simulink model "CS637Assignment3_1"  (R2022a)
settings: Solver=VariableStepAuto  StartTime=0.0  StopTime=5.0  RelTol=1e-3
model workspace (MAT data in the model file):
  I = 3.88e-07
  Kb = 0.000275
  Kt = 0.0059
  L = 0.00011
  R = 1.71
  b = 0
settings Model: Creator=kaush  LastModifiedBy=kaush

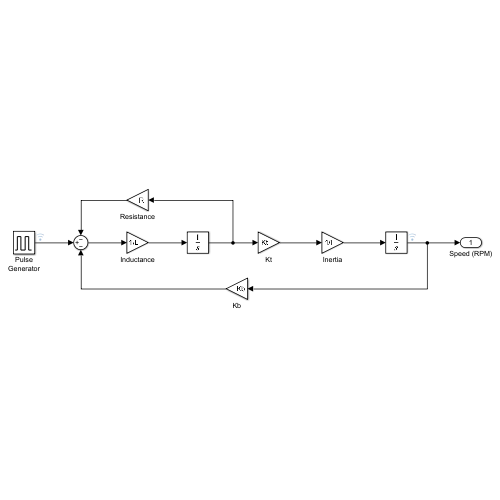
[thumbnail: Simulink's stored preview of the top-level diagram]
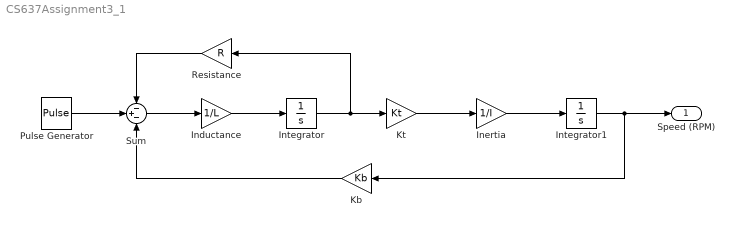
== system CS637Assignment3_1 ==
  Inductance : Gain  Gain=1/L
  Inertia : Gain  Gain=1/I
  Integrator : Integrator
  Integrator1 : Integrator
  Kb : Gain  Gain=Kb
  Kt : Gain  Gain=Kt
  Pulse Generator : DiscretePulseGenerator  PulseType=Time based  Period=0.001  PulseWidth=10
  Resistance : Gain  Gain=R
  Sum : Sum  Inputs=-+-
  Speed (RPM) : Outport
  wires:
  Kt/1 -> Inertia/1
  Inertia/1 -> Integrator1/1
  Sum/1 -> Inductance/1
  Inductance/1 -> Integrator/1
  Integrator1/1 -> Speed (RPM)/1, Kb/1
  Integrator/1 -> Kt/1, Resistance/1
  Kb/1 -> Sum/3
  Resistance/1 -> Sum/1
  Pulse Generator/1 -> Sum/2
